simulink model "Sl_H_Infinity_Close_loop"  (Simulink 8.5)
settings: Solver=ode45  StartTime=0.0  StopTime=10.0  RelTol=1e-3
libraries: cstblocks x2
settings Model: Creator=jordan  LastModifiedBy=Vladislav  CovSFcnEnable=off
settings DebuggingCC: SolverPrmCheckMsg=warning  FcnCallInpInsideContextMsg=UseLocalSettings

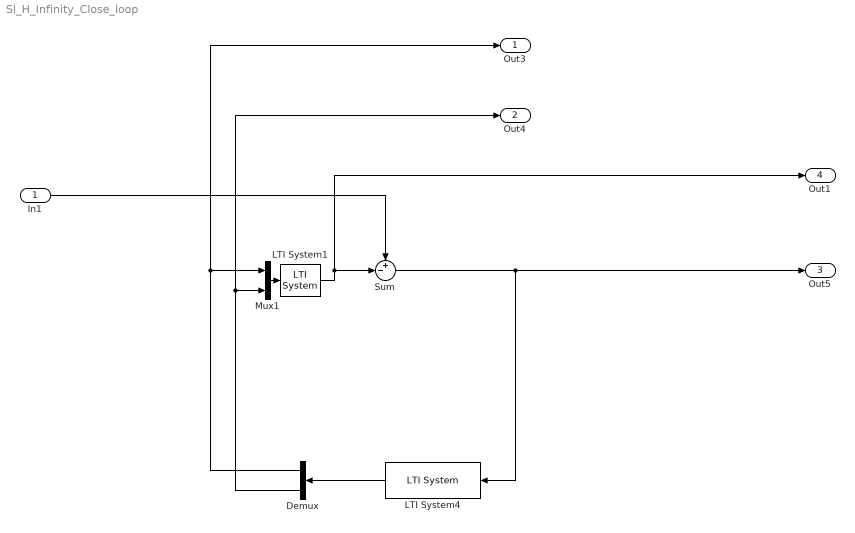
== system Sl_H_Infinity_Close_loop ==
  In1 : Inport
  Demux : Demux  Outputs=2
  LTI System1 : cstblocks/LTI System  sys=G  IC=[]
  LTI System4 : cstblocks/LTI System  sys=K  IC=[]
  Mux1 : Mux  Inputs=2
  Sum : Sum  Inputs=+-|
  Out3 : Outport
  Out4 : Outport  Port=2
  Out5 : Outport  Port=3
  Out1 : Outport  Port=4
  wires:
  LTI System1/1 -> Out1/1, Sum/2
  Sum/1 -> Out5/1, LTI System4/1
  In1/1 -> Sum/1
  LTI System4/1 -> Demux/1
  Demux/1 -> Mux1/1, Out3/1
  Demux/2 -> Mux1/2, Out4/1
  Mux1/1 -> LTI System1/1
